simulink model "VV_Jordan"  (R2018b)
settings: Solver=VariableStepAuto  StartTime=0.0  StopTime=10.0  RelTol=1e-3
settings Model: Creator=kekos  LastModifiedBy=kekos

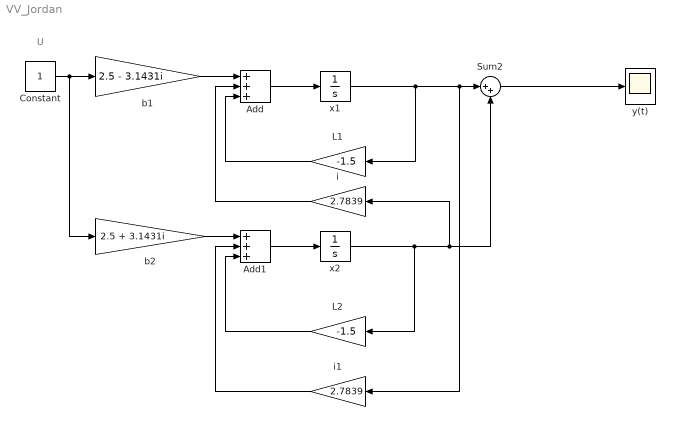
== system VV_Jordan ==
  note: U
  Add : Sum  Inputs=3
  Add1 : Sum  Inputs=3
  Constant : Constant
  L1 : Gain  Gain=-1.5
  L2 : Gain  Gain=-1.5
  Sum2 : Sum  Inputs=|++
  b1 : Gain  Gain=2.5 - 3.1431i
  b2 : Gain  Gain=2.5 + 3.1431i
  i : Gain  Gain=2.7839
  i1 : Gain  Gain=2.7839
  x1 : Integrator  InitialCondition=1
  x2 : Integrator  InitialCondition=1
  y(t) : Scope
  wires:
  b1/1 -> Add/1
  L1/1 -> Add/3
  i1/1 -> Add1/2
  Add/1 -> x1/1
  L2/1 -> Add1/3
  Constant/1 -> b2/1, b1/1
  Sum2/1 -> y(t)/1
  i/1 -> Add/2
  x1/1 -> L1/1, Sum2/1, i1/1
  x2/1 -> L2/1, Sum2/2, i/1
  b2/1 -> Add1/1
  Add1/1 -> x2/1
